simulink model "blockdemo"  (Simulink 6.3)
settings: Solver=FixedStepDiscrete  StartTime=0.0  StopTime=10.0  FixedStep=1  RelTol=1e-3
InitFcn:
  | %% DSPBuilder Start
  | alt_dspbuilder_update_model(bdroot)
  | %% DSPBuilder End
libraries: allblocks_alteradspbuilder2 x8
settings Model: LastModifiedBy=delphick

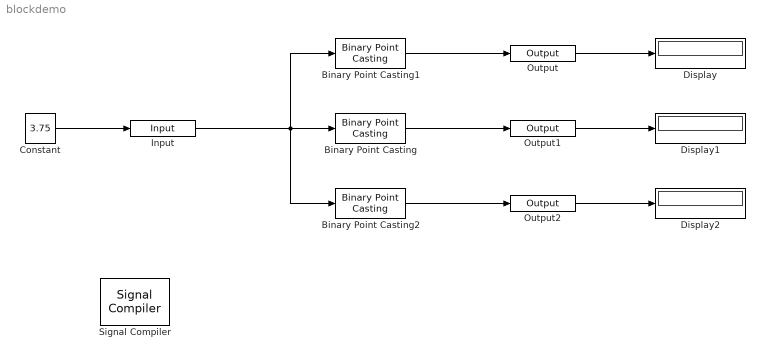
== system blockdemo ==
  Binary Point Casting : allblocks_alteradspbuilder2/Binary Point Casting  BusType=Signed Fractional  bwl=8  bwr=8  OutputPointPosition=8
  Binary Point Casting1 : allblocks_alteradspbuilder2/Binary Point Casting  BusType=Signed Fractional  bwl=8  bwr=8  OutputPointPosition=10
  Binary Point Casting2 : allblocks_alteradspbuilder2/Binary Point Casting  BusType=Signed Fractional  bwl=8  bwr=8  OutputPointPosition=4
  Constant : Constant  Value=3.75
  Display : Display
  Display1 : Display
  Display2 : Display
  Input : allblocks_alteradspbuilder2/Input  iofile=C:\workspace_clean\Documentation\DesignExamples\Tutorials\UnitBlocks\IOBus\BPC\tb_blockdemo\blockdemo_Input.salt  BusType=Signed Fractional  bwl=8  bwr=8  SpecifyClock=off  PORTTYPE=Input
  Output : allblocks_alteradspbuilder2/Output  iofile=C:\workspace_clean\Documentation\DesignExamples\Tutorials\UnitBlocks\IOBus\BPC\tb_blockdemo\blockdemo_Output.capture  BusType=Inferred  bwl=8  bwr=0  PORTTYPE=Output
  Output1 : allblocks_alteradspbuilder2/Output  iofile=C:\workspace_clean\Documentation\DesignExamples\Tutorials\UnitBlocks\IOBus\BPC\tb_blockdemo\blockdemo_Output1.capture  BusType=Inferred  bwl=8  bwr=0  PORTTYPE=Output
  Output2 : allblocks_alteradspbuilder2/Output  iofile=C:\workspace_clean\Documentation\DesignExamples\Tutorials\UnitBlocks\IOBus\BPC\tb_blockdemo\blockdemo_Output2.capture  BusType=Inferred  bwl=8  bwr=0  PORTTYPE=Output
  Signal Compiler : allblocks_alteradspbuilder2/Signal Compiler  DeviceFamily=Stratix IV  DeviceName=AUTO  EnableSignalTap=off  SignalTapDepth=128  UseBoardBlock=off  StpUseDefaultClock=on  StpClock=clock
  wires:
  Constant/1 -> Input/1
  Input/1 -> Binary Point Casting/1, Binary Point Casting1/1, Binary Point Casting2/1
  Binary Point Casting1/1 -> Output/1
  Binary Point Casting/1 -> Output1/1
  Binary Point Casting2/1 -> Output2/1
  Output/1 -> Display/1
  Output1/1 -> Display1/1
  Output2/1 -> Display2/1
